simulink model "TMsimulation2018a"  (R2018a)
settings: Solver=VariableStepDiscrete  StartTime=0.0  StopTime=inf  RelTol=1e-3
values from neighbouring files (symbols this model uses):
  atmoLoss = 0.501    [modelParameters.m]
  cableLossG = 0.501    [modelParameters.m]
  Grx = 10000    [modelParameters.m]
  Gtx = 19.275    [modelParameters.m]
  lna = 1    [modelParameters.m]
  pointingLossG = 0.891    [modelParameters.m]
  pointingLossOB = 0.999    [modelParameters.m]
  polarizationLossOB = 0.776    [modelParameters.m]
undefined symbols (not defined in the file or in its folder): comm, constellation, rsgenpoly
libraries: commblkcod2 x2, commcnvcod2 x2, commrflib2 x2, commblkintrlv2 x2, commdigbbndpm3 x2, commrandsrc3 x1, commsink2 x1, commutil2 x1
settings Model: Creator=Michele Genoni  LastModifiedBy=Michele Genoni
settings DataIOCC: LimitDataPoints=on  SaveOutput=off  SaveTime=off
settings OptimizationCC: BooleanDataType=off  DefaultParameterBehavior=Inlined  LocalBlockOutputs=off  LifeSpan=inf
settings DebuggingCC: AlgebraicLoopMsg=error  SingleTaskRateTransMsg=error  AllowSymbolicDim=off  SFUnexpectedBacktrackingDiag=warning  SFNoUnconditionalDefaultTransitionDiag=warning  SFExecutionAtInitializationDiag=none
settings CodeAppCC: StateflowObjectComments=on
settings GRTTargetCC: TargetLangStandard=C89/C90 (ANSI)  GeneratePreprocessorConditionals=Disable all
settings ConfigComp: CovMetricSettings=dw  CovHtmlReporting=on  CovSaveCumulativeToWorkspaceVar=on  CovSaveSingleToWorkspaceVar=on  CovExternalEMLEnable=off  CovSFcnEnable=off

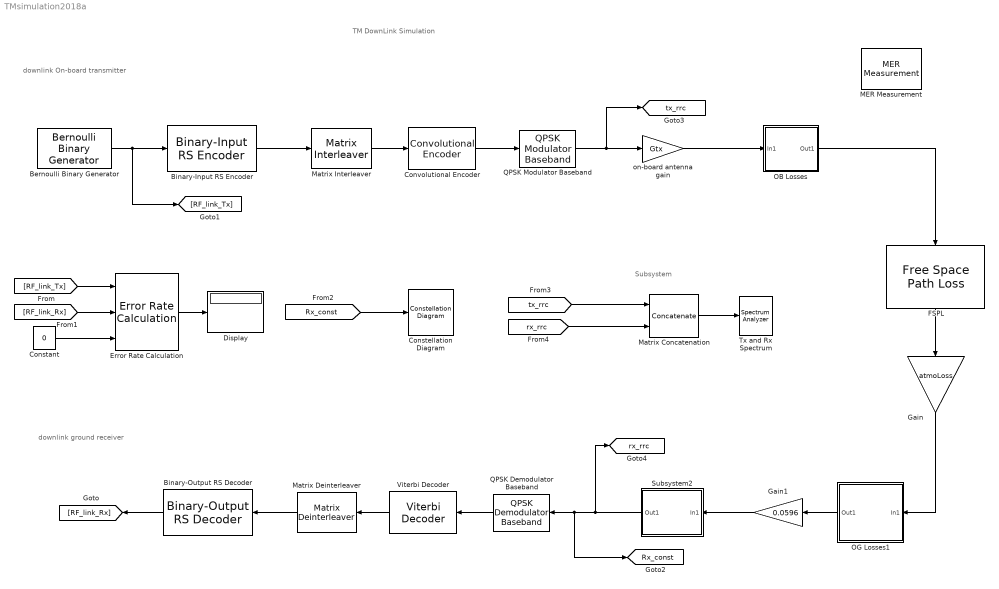
== system TMsimulation2018a ==
  note: Subsystem
  note: downlink On-board transmitter
  note: TM DownLink Simulation
  note: downlink ground receiver
  Bernoulli Binary Generator : commrandsrc3/Bernoulli Binary Generator  ProbabilityOfZero=0.5  SeedSource=Auto  Seed=0  SampleTime=4.0832*10^-8  SamplesPerFrame=223*5*8  OutputDataType=double  SimulateUsing=Interpreted execution
  Binary-Input RS Encoder : commblkcod2/Binary-Input RS Encoder  n=255  k=223  specShortening=off  shortenedK=3  specGenPoly=off  genPoly=rsgenpoly(7, 3, [], [], 'double')  specPrimPoly=off  prPoly='X^3 + X + 1'  specPuncture=off  punctVec=[ones(2,1); zeros(2,1)]  outDType=Same as input
      settings: SourceProductName=Communications System Toolbox  SourceProductBaseCode=CM
  Binary-Output RS Decoder : commblkcod2/Binary-Output RS Decoder  n=255  k=223  specShortening=off  shortenedK=3  specGenPoly=off  genPoly=rsgenpoly(7, 3, [], [], 'double')  specPrimPoly=off  prPoly='X^3 + X + 1'  specPuncture=off  punctVec=[ones(2,1); zeros(2,1)]  specErasurePort=off  showNumErr=off  outDType=Same as input
      settings: SourceProductName=Communications System Toolbox  SourceProductBaseCode=CM
  Constant : Constant  Value=0
  Constellation Diagram : ConstellationDiagram
  Convolutional Encoder : commcnvcod2/Convolutional Encoder  trellis=poly2trellis(7, [171 133],171)  opMode=Truncated (reset every frame)  DelayedResetAction=off  hasIniStPort=off  hasFinStPort=off  usePuncVector=off  punctureVector=[1; 1; 0; 1; 0; 1]  reset=Unused parameter value
      settings: SourceProductName=Communications System Toolbox  SourceProductBaseCode=CM
  Display : Display
      settings: Format=short_e
  Error Rate Calculation : commsink2/Error Rate Calculation  N=0  st_delay=0  cp_mode=Entire frame  subframe=[]  PMode=Port  WsName=ErrorVec  RsMode2=on  stop=off  numErr=100  maxBits=1e6
  "FSPL " : commrflib2/Free Space Path Loss  mode=Decibels  dB=178  d=0.100  fc=1920
      settings: SourceProductName=Communications System Toolbox  SourceProductBaseCode=CM
  Gain : Gain  Gain=atmoLoss
  Gain1 : Gain  Gain=0.0596
  MER Measurement : commutil2/MER Measurement  ReferenceSignalSource=Input port  ReferenceConstellation=constellation( comm.QPSKModulator )  MeasurementIntervalSource=Input length  MeasurementInterval=100  AveragingDimensions=1  MinimumMEROutputPort=off  XPercentileMEROutputPort=off  XPercentileValue=95  SymbolCountOutputPort=off  SimulateUsing=Interpreted execution
      settings: SourceProductName=Communications System Toolbox  SourceProductBaseCode=CM
  Matrix Concatenation : Concatenate  Mode=Multidimensional array  ConcatenateDimension=2
  Matrix Deinterleaver : commblkintrlv2/Matrix Deinterleaver  Nrows=5  Ncols=255*8
      settings: SourceProductName=Communications System Toolbox  SourceProductBaseCode=CM
  Matrix Interleaver : commblkintrlv2/Matrix Interleaver  Nrows=5  Ncols=255*8
      settings: SourceProductName=Communications System Toolbox  SourceProductBaseCode=CM
  OB Losses : Subsystem
  OG Losses1 : Subsystem
  QPSK Demodulator Baseband : commdigbbndpm3/QPSK Demodulator Baseband  OutType=Bit  DecType=Hard decision  VarSource=Dialog  Variance=1  Dec=Gray  Ph=pi/4  outDtype1=Inherit via internal rule  outDtype2=Inherit via internal rule  derotateFactorWordLen=16  derotateFactorDataTypeStr=Inherit: Same word length as input  derotateFactorLastDataTypeStr=Inherit: Same word length as input
  QPSK Modulator Baseband : commdigbbndpm3/QPSK Modulator Baseband  InType=Bit  Enc=Gray  Ph=pi/4  outDtype=double  outWordLen=16  outUDDataType=sfix(16)  outFracLenMode=Best precision  outFracLen=15  outDataTypeStr=double  outLastDataTypeStr=double
  Subsystem2 : Subsystem
      mask Display: disp('receiving \n antenna')
  Tx and Rx Spectrum : SpectrumAnalyzer
  Viterbi Decoder : commcnvcod2/Viterbi Decoder  trellis=poly2trellis(7, [171 133],171)  isPunctured=off  punctureVector=[1; 1; 0; 1; 0; 1]  erasures=off  dectype=Hard decision  nsdecb=4  runSigValErrCheck=off  tbdepth=34  opmode=Truncated  reset=off  delayedResetAction=off  smWordLength=16  outDataType=Inherit via internal rule
      settings: SourceProductName=Communications System Toolbox  SourceProductBaseCode=CM
  on-board antenna gain : Gain  Gain=Gtx
  tag scope: Rx_const=global, rx_rrc=global, tx_rrc=global
  wires:
  Bernoulli Binary Generator/1 -> Binary-Input RS Encoder/1, [RF_link_Tx]
  Binary-Output RS Decoder/1 -> [RF_link_Rx]
  [Rx_const] -> Constellation Diagram/1
  QPSK Modulator Baseband/1 -> [tx_rrc], on-board antenna gain/1
  Error Rate Calculation/1 -> Display/1
  Subsystem2/1(Out1) -> [Rx_const], QPSK Demodulator Baseband/1, [rx_rrc]
  "FSPL "/1 -> Gain/1
  [RF_link_Tx] -> Error Rate Calculation/1
  [RF_link_Rx] -> Error Rate Calculation/2
  [rx_rrc] -> Matrix Concatenation/2
  [tx_rrc] -> Matrix Concatenation/1
  Matrix Concatenation/1 -> Tx and Rx Spectrum/1
  on-board antenna gain/1 -> OB Losses/1(In1)
  Gain/1 -> OG Losses1/1(In1)
  OG Losses1/1(Out1) -> Gain1/1
  Gain1/1 -> Subsystem2/1(In1)
  Constant/1 -> Error Rate Calculation/3
  Binary-Input RS Encoder/1 -> Matrix Interleaver/1
  Matrix Deinterleaver/1 -> Binary-Output RS Decoder/1
  QPSK Demodulator Baseband/1 -> Viterbi Decoder/1
  Matrix Interleaver/1 -> Convolutional Encoder/1
  Convolutional Encoder/1 -> QPSK Modulator Baseband/1
  Viterbi Decoder/1 -> Matrix Deinterleaver/1
  OB Losses/1(Out1) -> "FSPL "/1

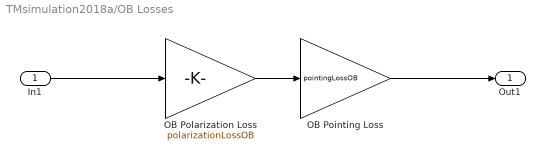
== system TMsimulation2018a/OB Losses ==
  In1 : Inport
  OB Pointing Loss : Gain  Gain=pointingLossOB
  OB Polarization Loss : Gain  Gain=polarizationLossOB
  Out1 : Outport
  wires:
  OB Polarization Loss/1 -> OB Pointing Loss/1
  In1/1 -> OB Polarization Loss/1
  OB Pointing Loss/1 -> Out1/1

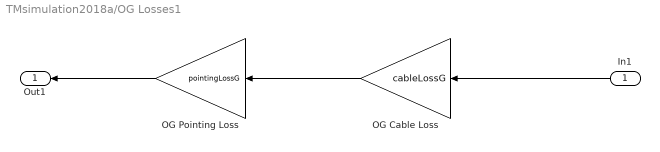
== system TMsimulation2018a/OG Losses1 ==
  In1 : Inport
  OG Cable Loss : Gain  Gain=cableLossG
  OG Pointing Loss : Gain  Gain=pointingLossG
  Out1 : Outport
  wires:
  OG Pointing Loss/1 -> Out1/1
  In1/1 -> OG Cable Loss/1
  OG Cable Loss/1 -> OG Pointing Loss/1

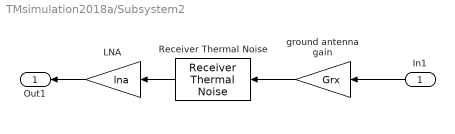
== system TMsimulation2018a/Subsystem2 ==
  In1 : Inport
  LNA : Gain  Gain=lna
  Receiver Thermal Noise : commrflib2/Receiver Thermal Noise  method=Noise figure  ntemp=35  nfigure=noiseFigure  nfactor=2  add290KAntennaNoise=off  seed=67987
      settings: SourceProductName=Communications System Toolbox  SourceProductBaseCode=CM
  ground antenna gain : Gain  Gain=Grx
  Out1 : Outport
  wires:
  ground antenna gain/1 -> Receiver Thermal Noise/1
  In1/1 -> ground antenna gain/1
  Receiver Thermal Noise/1 -> LNA/1
  LNA/1 -> Out1/1
